simulink model "FIR_TDM_FirstPrinciples"  (R2024a)
settings: Solver=VariableStepAuto  StartTime=0.0  StopTime=inf  RelTol=1e-3
InitFcn:
  | SamplesPerChannel = 2;
  | NumOf_TDM_Channels = 4;
  | FilterLength = 4;
  | filters = reshape(complex(1:(FilterLength*NumOf_TDM_Channels), 1:(FilterLength*NumOf_TDM_Channels)), FilterLength, NumOf_TDM_Channels);
undefined symbols (not defined in the file): Asymmetric, S, vsva2197, xcvc1902
libraries: aieDSP x1, dspobslib x1, dspsrcs4 x1, aieUtilities x1, vmcUtilities x1
settings Model: Creator=sdegala  LastModifiedBy=robg
settings RTWCC: GPUComputeCapability=3.5

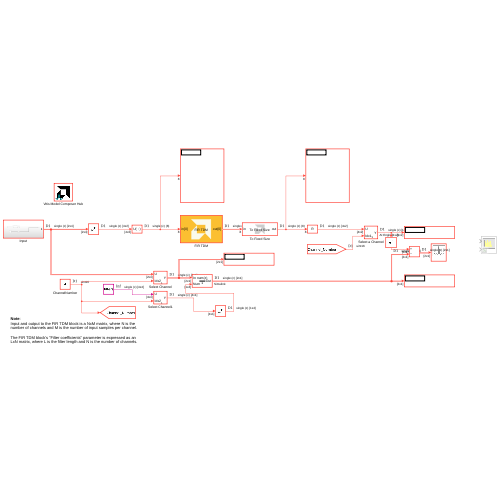
[thumbnail: Simulink's stored preview of the top-level diagram]
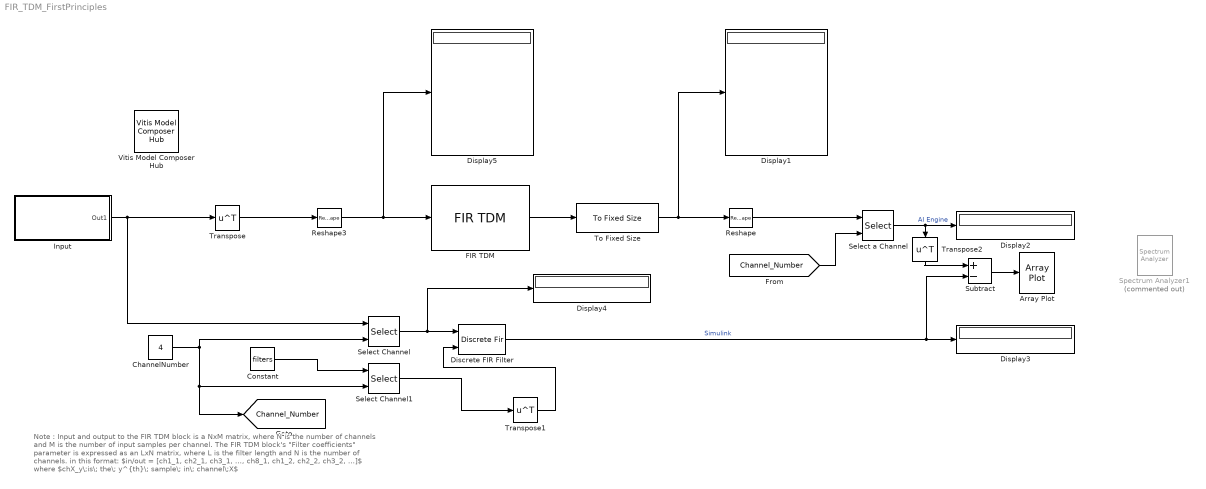
== system FIR_TDM_FirstPrinciples ==
  note: Note :
      | Input and output to the FIR TDM block is a NxM matrix, where N is the number of channels and M is the number of input samples per channel.
      |
      | The FIR TDM block's "Filter coefficients" parameter is expressed as an LxN matrix, where L is the filter length and N is the number of channels.
      |
      | in this format:
      |
      | $in/out = [ch1_1, ch2_1, ch3_1, ..., ch8_1, ch1_2, ch2_2, ch3_2, ...]$
      |
      | where $chX_y\;is\; the\; y^{th}\; sample\; in\; channel\;X$
  Array Plot : ArrayPlot  WindowPosition=[1626.000000,639.000000,800.000000,500.000000,]  Visible=on  ScopeFrameLocation=window  PlotType=Line  YLimits=[-1.3059 1.4328]  ShowLegend=on
  ChannelNumber : Constant  Value=4  OutDataTypeStr=uint16  SampleTime=-1
  Constant : Constant  Value=filters  OutDataTypeStr=single
  Discrete FIR Filter : DiscreteFir  CoefSource=Input port  Coefficients=(1:4)+1i*(1:4)  InputProcessing=Columns as channels (frame based)  RndMeth=Round
      settings: InputPortMap=u0,u1
  Display{1..5} (5 alike) : Display
  FIR TDM : aieDSP/FIR TDM  data_type=cfloat  data_out_type=cfloat  coef_type=cfloat  fir_length=FilterLength  coeff=filters  shift_val=0  rnd_mode=Floor  input_window_size=SamplesPerChannel*NumOf_TDM_Channels  tdm_channels=NumOf_TDM_Channels  sat_mode=1-Asymmetric  casc_length=1  ssr=1  AIE_VARIANT=1  blockJsonConstraints=[]  blockJsonConstraintsInternal=[]  spec=vmc_fir_tdm.json  SerializedMaskParamNames=[]  SerializedMaskParamValues=[]  SerializedMaskParamVisibilities=[]  block_type=FIR TDM  SerializedMaskParamDataypes=typename|typename|typename|uint|coef_type|uint|uint|uint|uint|uint|uint|uint|uint  SerializedMaskParamEnumStrArr=0|0|0|0|0|0|Floor,Ceiling,Round to positive infinity,Round to negative infinity,Round symmetrical to infinity,Round symmetrical to zero,Round convergent to even,Round convergent to odd|0|0|0-None,1-Asymmetric,3-Symmetric|0|0|0  SerializedMaskParamEnumValArr=0|0|0|0|0|0|0,1,2,3,4,5,6,7|0|0|0,1,3|0|0|0  SerializedMaskParamVectorArr=0|0|0|0|1|0|0|0|0|0|0|0|0
  Input : Subsystem
  Reshape : Reshape  OutputDimensionality=Customize  OutputDimensions=[NumOf_TDM_Channels,SamplesPerChannel]
  Reshape3 : Reshape
  Select Channel : Selector  NumberOfDimensions=2  InputPortWidth=3  IndexOptions=Select all,Index vector (port)  Indices=3,[16]  OutputSizes=1,1
  Select Channel1 : Selector  NumberOfDimensions=2  InputPortWidth=3  IndexOptions=Select all,Index vector (port)  Indices=3,[16]  OutputSizes=1,1
  Select a Channel : Selector  NumberOfDimensions=2  InputPortWidth=3  IndexOptions=Index vector (port),Select all  Indices=3,[16]  OutputSizes=1,1
  Spectrum Analyzer1 : SpectrumAnalyzer  Commented=on  NumInputPorts=2  WindowPosition=[1529.000000,30.000000,936.000000,716.000000,]  ScopeFrameLocation=window  Span=12499.999999999998  StartFrequency=-6249.999999999999  StopFrequency=6249.999999999999  YLimits=[-104.13003505,11.17463747]  ShowLegend=on  MeasurementChannel=2
      settings: OpenAtSimulationStart=off
  Subtract : Sum  Inputs=+-
  To Fixed Size : aieUtilities/To Fixed Size  Mode=Stop simulation when input variable-size signal is not full  OutputSize=Inherit: Same as input  CopyMethod=Buffer samples to form output  HasStatusOutput=on
  Transpose : Math  Operator=transpose
  Transpose1 : Math  Operator=transpose
  Transpose2 : Math  Operator=transpose
  Vitis Model Composer Hub : vmcUtilities/Vitis Model Composer Hub  Tag=genX  CodeGeneration=off  StartColumn=1  NumberOfColumns=1  TargetDirectory=./code  exportDesign=off  analyzeDesign=off  validateDesignOnHw=off  ExportType=AI Engines  IpVendor=xilinx.com  IpLibrary=hls  IpVersion=1.0  IpHWLanguage=Verilog  AieCompilerOptions={}  AieSimulatorOptions={}  CreateTestbench=off  TestbenchStackSize=10  RunRtlSim=off  RunCSim=off  RunAieSim=off  AieSimTimeout=50000  RunAieSimProfiling=off  LaunchVitisAnalyzer=off  PlotOutput=off  RunX86Sim=off  X86SimTimeout=10  GenHwImage=off  GenLibadfXo=off  GenHwValidationCode=off  PlatformType=Not Specified  HwSystemType=Baremetal  HwValidationTarget=hw  ProjDevice=xcvc1902-vsva2197-1LP-e-S  ProjDevicePart=xcvc1902-vsva2197-1LP-e-S  AIEType=AIE  SamplePeriod=-1  ClockFrequency=200  DataPathParallelism=1  xilinxfamily=versalaicore  part=xcvc1902  speed=-1LP-e-S  package=vsva2197  directory=./netlist  testbench=off  incr_netlist=off  synthesis_tool=Vivado  clock_wrapper=Clock Enables  dbl_ovrd=According to Block Masks  dcm_input_clock_period=10  sysclk_period=10  simulink_period=1  eval_field=0  LogFileName=''  NThreads=4
  tag scope: Channel_Number=global
  wires:
  Select a Channel/1 -> Transpose2/1, Display2/1  "AI Engine"
  Discrete FIR Filter/1 -> Subtract/2, Display3/1  "Simulink"
  Select Channel/1 -> Display4/1, Discrete FIR Filter/1
  ChannelNumber/1 -> Select Channel1/2, [Channel_Number], Select Channel/2
  [Channel_Number] -> Select a Channel/2
  Reshape3/1 -> Display5/1, FIR TDM/1
  FIR TDM/1 -> To Fixed Size/1
  Subtract/1 -> Array Plot/1
  To Fixed Size/1 -> Reshape/1, Display1/1
  Reshape/1 -> Select a Channel/1
  Constant/1 -> Select Channel1/1
  Select Channel1/1 -> Transpose1/1
  Transpose1/1 -> Discrete FIR Filter/2
  Transpose2/1 -> Subtract/1
  Input/1(Out1) -> Transpose/1, Select Channel/1
  Transpose/1 -> Reshape3/1

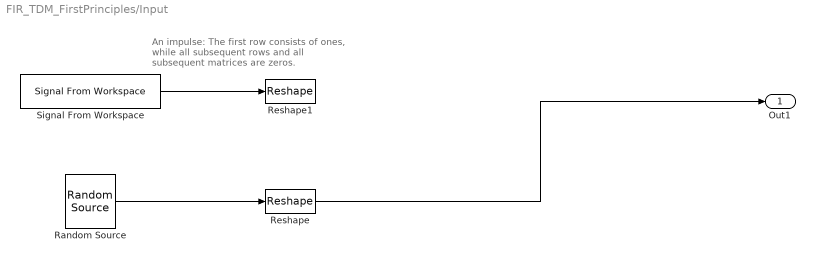
== system FIR_TDM_FirstPrinciples/Input ==
  note: An impulse: The first row consists of ones,
      | while all subsequent rows and all subsequent matrices are zeros.
  Random Source : dspobslib/Random Source  SrcType=Gaussian  NormMethod=Ziggurat  CltLength=12  MinVal=0  MaxVal=1  MeanVal=0  VarVal=1e-4  RepMode=Specify seed  rawSeed=1  IsInherit=off  SampMode=Discrete  SampTime=1/100e3  SampFrame=SamplesPerChannel*NumOf_TDM_Channels  DataType=Single  OutComplex=Complex  OutputFrames=on
  Reshape : Reshape  OutputDimensionality=Customize  OutputDimensions=[SamplesPerChannel,NumOf_TDM_Channels]
  Reshape1 : Reshape  OutputDimensionality=Customize  OutputDimensions=[SamplesPerChannel,NumOf_TDM_Channels]
  Signal From Workspace : dspsrcs4/Signal From Workspace  X=complex(single(ones(1,NumOf_TDM_Channels)))  Ts=1/100e3  nsamps=SamplesPerChannel*NumOf_TDM_Channels  OutputAfterFinalValue=Setting to zero  ignoreOrWarnInputAndFrameLengths=off  OutputFrames=off
  Out1 : Outport
  wires:
  Random Source/1 -> Reshape/1
  Signal From Workspace/1 -> Reshape1/1
  Reshape/1 -> Out1/1
